simulink model "HT07PowertrainThermalModel3"  (R2022b)
(part 2 of 2)

  PS Gain : fl_lib/Physical Signals/Functions/PS Gain  gain=1
  PS Gain1 : fl_lib/Physical Signals/Functions/PS Gain  gain=2
  PS Gain2 : fl_lib/Physical Signals/Functions/PS Gain  gain=1
  PS Lookup Table (1D) : fl_lib/Physical Signals/Lookup Tables/PS Lookup Table (1D)  x=time  f=motorRearHeatGen J/s  interp_method=simscape.enum.interpolation.linear  extrap_method=simscape.enum.extrapolation.nearest
  PS Lookup Table (1D)1 : fl_lib/Physical Signals/Lookup Tables/PS Lookup Table (1D)  x=time  f=mcuHeatGen J/s  interp_method=simscape.enum.interpolation.linear  extrap_method=simscape.enum.extrapolation.nearest
  PS Lookup Table (1D)2 : fl_lib/Physical Signals/Lookup Tables/PS Lookup Table (1D)  x=time  f=velocity m/s  interp_method=simscape.enum.interpolation.linear  extrap_method=simscape.enum.extrapolation.nearest
  PS Lookup Table (1D)3 : fl_lib/Physical Signals/Lookup Tables/PS Lookup Table (1D)  Commented=on  x=time  f=velocity m/s  interp_method=simscape.enum.interpolation.linear  extrap_method=simscape.enum.extrapolation.nearest
  PS Lookup Table (1D)6 : fl_lib/Physical Signals/Lookup Tables/PS Lookup Table (1D)  Commented=on  x=time  f=velocity m/s  interp_method=simscape.enum.interpolation.linear  extrap_method=simscape.enum.extrapolation.nearest
  PS Lookup Table (1D)7 : fl_lib/Physical Signals/Lookup Tables/PS Lookup Table (1D)  x=time  f=motorFrontHeatGen J/s  interp_method=simscape.enum.interpolation.linear  extrap_method=simscape.enum.extrapolation.nearest
  PS Product : fl_lib/Physical Signals/Functions/PS Product
  PS Product1 : fl_lib/Physical Signals/Functions/PS Product  Commented=on
  PS Product2 : fl_lib/Physical Signals/Functions/PS Product  Commented=on
  PS Ramp{,1..2,5} (4 alike) : fl_lib/Physical Signals/Sources/PS Ramp  slope=1 1/s  start_time=0 s  initial_output=0
  PS Ramp3 : fl_lib/Physical Signals/Sources/PS Ramp  Commented=on  slope=1 1/s  start_time=0 s  initial_output=0
  PS Ramp4 : fl_lib/Physical Signals/Sources/PS Ramp  Commented=on  slope=1 1/s  start_time=0 s  initial_output=0
  PS-Simulink Converter{,5..8,11,31} (7 alike) : nesl_utility/PS-Simulink Converter  PhysicalDomain=network_engine_domain  SubClassName=ps_output  LeftPortType=input  RightPortType=output  PseudoPeriodic=off  Frequencies=[]  VectorFormat=inherit  Unit=inherit  AffineConversion=off
  PS-Simulink Converter1 : nesl_utility/PS-Simulink Converter  PhysicalDomain=network_engine_domain  SubClassName=ps_output  LeftPortType=input  RightPortType=output  PseudoPeriodic=off  Frequencies=[]  VectorFormat=1-D array  Unit=inherit  AffineConversion=off
  PS-Simulink Converter{3,9..10,13..18,20..30} (20 alike) : nesl_utility/PS-Simulink Converter  Commented=on  PhysicalDomain=network_engine_domain  SubClassName=ps_output  LeftPortType=input  RightPortType=output  PseudoPeriodic=off  Frequencies=[]  VectorFormat=inherit  Unit=inherit  AffineConversion=off
  PS-Simulink Converter12 : nesl_utility/PS-Simulink Converter  Commented=on  PhysicalDomain=network_engine_domain  SubClassName=ps_output  LeftPortType=input  RightPortType=output  PseudoPeriodic=off  Frequencies=[]  VectorFormat=1-D array  Unit=inherit  AffineConversion=off
  PS-Simulink Converter19 : nesl_utility/PS-Simulink Converter  Commented=on  PhysicalDomain=network_engine_domain  SubClassName=ps_output  LeftPortType=input  RightPortType=output  PseudoPeriodic=off  Frequencies=[]  VectorFormat=1-D array  Unit=inherit  AffineConversion=off
  PS-Simulink Converter2 : nesl_utility/PS-Simulink Converter  PhysicalDomain=network_engine_domain  SubClassName=ps_output  LeftPortType=input  RightPortType=output  PseudoPeriodic=off  Frequencies=[]  VectorFormat=1-D array  Unit=inherit  AffineConversion=off
  PS-Simulink Converter4 : nesl_utility/PS-Simulink Converter  PhysicalDomain=network_engine_domain  SubClassName=ps_output  LeftPortType=input  RightPortType=output  PseudoPeriodic=off  Frequencies=[]  VectorFormat=1-D array  Unit=inherit  AffineConversion=off
  PUMP TO MCU : fl_lib/Thermal Liquid/Elements/Pipe (TL)  Commented=on  length=tubeLengthPumpToMCU m  area=A m^2  Dh=d m  length_add=leqMCUToMotor m  roughness=tubeRoughness m  Re_lam=2000  Re_tur=4000  shape_factor=64  Nu_lam=3.66  dynamic_compressibility=simscape.enum.onoff.off  inertia=simscape.enum.onoff.off  p0=0.101325 MPa  T0=Tambient degC  mdot0=0 kg/s
  Perfect Insulator{,1..2,5} (4 alike) : fl_lib/Thermal/Thermal Elements/Perfect Insulator  T_specify=off  T_priority=None  T=0 K  T_nominal_specify=off  T_nominal_unit=K  T_nominal_value=1
  Perfect Insulator10 : fl_lib/Thermal/Thermal Elements/Perfect Insulator  Commented=on  T_specify=on  T_priority=High  T=Tambient degC  T_nominal_specify=off  T_nominal_unit=degC  T_nominal_value=Tambient
  Perfect Insulator12 : fl_lib/Thermal/Thermal Elements/Perfect Insulator  Commented=on  T_specify=off  T_priority=None  T=293.15 K  T_nominal_specify=off  T_nominal_unit=K  T_nominal_value=1
  Perfect Insulator13 : fl_lib/Thermal/Thermal Elements/Perfect Insulator  Commented=on  T_specify=off  T_priority=None  T=293.15 K  T_nominal_specify=off  T_nominal_unit=K  T_nominal_value=1
  Perfect Insulator14 : fl_lib/Thermal/Thermal Elements/Perfect Insulator  Commented=on  T_specify=off  T_priority=None  T=293.15 K  T_nominal_specify=off  T_nominal_unit=K  T_nominal_value=1
  Perfect Insulator{3,6,8..9} (4 alike) : fl_lib/Thermal/Thermal Elements/Perfect Insulator  Commented=on  T_specify=off  T_priority=None  T=0 K  T_nominal_specify=off  T_nominal_unit=K  T_nominal_value=1
  Perfect Insulator7 : fl_lib/Thermal/Thermal Elements/Perfect Insulator  Commented=on  T_specify=on  T_priority=High  T=Tambient degC  T_nominal_specify=off  T_nominal_unit=degC  T_nominal_value=Tambient
  Pipe (TL)1 : fl_lib/Thermal Liquid/Elements/Pipe (TL)  length=tubeLengthRadiatorToPump m  area=A m^2  Dh=d m  length_add=0 m  roughness=tubeRoughness m  Re_lam=2000  Re_tur=4000  shape_factor=64  Nu_lam=3.66  dynamic_compressibility=simscape.enum.onoff.off  inertia=simscape.enum.onoff.off  p0=0.101325 MPa  T0=Tamb degC  mdot0=0 kg/s
  Pipe (TL)2 : fl_lib/Thermal Liquid/Elements/Pipe (TL)  Commented=on  length=350 mm  area=A m^2  Dh=d m  length_add=0 m  roughness=tubeRoughness m  Re_lam=2000  Re_tur=4000  shape_factor=64  Nu_lam=3.66  dynamic_compressibility=simscape.enum.onoff.off  inertia=simscape.enum.onoff.off  p0=0.101325 MPa  T0=Tambient degC  mdot0=0 kg/s
  Pipe (TL)3 : fl_lib/Thermal Liquid/Elements/Pipe (TL)  length=tubeLengthMCUToMotor m  area=A m^2  Dh=d m  length_add=leqMCUToMotor m  roughness=tubeRoughness m  Re_lam=2000  Re_tur=4000  shape_factor=64  Nu_lam=3.66  dynamic_compressibility=simscape.enum.onoff.off  inertia=simscape.enum.onoff.off  p0=0.101325 MPa  T0=Tamb degC  mdot0=0 kg/s
  Pipe (TL)4 : fl_lib/Thermal Liquid/Elements/Pipe (TL)  length=tubeLengthMotorToRadiator m  area=A m^2  Dh=d m  length_add=leqMotorToRadiator m  roughness=tubeRoughness m  Re_lam=2000  Re_tur=4000  shape_factor=64  Nu_lam=3.66  dynamic_compressibility=simscape.enum.onoff.off  inertia=simscape.enum.onoff.off  p0=0.101325 MPa  T0=Tamb degC  mdot0=0 kg/s
  Pipe (TL)5 : fl_lib/Thermal Liquid/Elements/Pipe (TL)  length=tubeLengthPumpToMCU m  area=A m^2  Dh=d m  length_add=leqMCUToMotor m  roughness=tubeRoughness m  Re_lam=2000  Re_tur=4000  shape_factor=64  Nu_lam=3.66  dynamic_compressibility=simscape.enum.onoff.off  inertia=simscape.enum.onoff.off  p0=0.101325 MPa  T0=Tamb degC  mdot0=0 kg/s
  Pipe (TL)6 : fl_lib/Thermal Liquid/Elements/Pipe (TL)  Commented=on  length=210 mm  area=pi*((3/4)^2)/4 in^2  Dh=3/4 in  length_add=0 m  roughness=tubeRoughness m  Re_lam=2000  Re_tur=4000  shape_factor=64  Nu_lam=3.66  dynamic_compressibility=simscape.enum.onoff.off  inertia=simscape.enum.onoff.off  p0=0.101325 MPa  T0=Tambient degC  mdot0=0 kg/s
  Pipe (TL)7 : fl_lib/Thermal Liquid/Elements/Pipe (TL)  Commented=on  length=115 mm  area=pi*(0.5^2)/4 m^2  Dh=0.5 in  length_add=0 m  roughness=tubeRoughness m  Re_lam=2000  Re_tur=4000  shape_factor=64  Nu_lam=3.66  dynamic_compressibility=simscape.enum.onoff.off  inertia=simscape.enum.onoff.off  p0=0.101325 MPa  T0=Tambient degC  mdot0=0 kg/s
  Pressure & Temperature Sensor (TL){1..2,4..6,20} (6 alike) : fl_lib/Thermal Liquid/Sensors/Pressure & Temperature Sensor (TL)
      settings: InternalSimscapePortConfiguration="{\"Bottom\":[],\"Left\":[{\"id\":\"A\",\"label\":\"A\",\"type\":\"foundation.thermal_liquid.thermal_liquid\"}],\"Right\":[{\"id\":\"B\",\"label\":\"B\",\"type\":\"foundation.thermal_liquid.thermal_liquid\"},{\"id\":\"P\",\"label\":\"P\",\"type\":\"output\"},{\"id\":\"T\",\"label\":\"T\",\"type\":\"output\"}],\"Top\":[]}"
  Pressure & Temperature Sensor (TL){3,7..19} (14 alike) : fl_lib/Thermal Liquid/Sensors/Pressure & Temperature Sensor (TL)  Commented=on
      settings: InternalSimscapePortConfiguration="{\"Bottom\":[],\"Left\":[{\"id\":\"A\",\"label\":\"A\",\"type\":\"foundation.thermal_liquid.thermal_liquid\"}],\"Right\":[{\"id\":\"B\",\"label\":\"B\",\"type\":\"foundation.thermal_liquid.thermal_liquid\"},{\"id\":\"P\",\"label\":\"P\",\"type\":\"output\"},{\"id\":\"T\",\"label\":\"T\",\"type\":\"output\"}],\"Top\":[]}"
  Pressure Drop Across Pump : nesl_utility/PS-Simulink Converter  PhysicalDomain=network_engine_domain  SubClassName=ps_output  LeftPortType=input  RightPortType=output  PseudoPeriodic=off  Frequencies=[]  VectorFormat=1-D array  Unit=inherit  AffineConversion=off
  Pressures : Scope
  Product : Product
  Product1 : Product  Commented=on
  Product3 : Product  Commented=on
  RADIATOR TO SENSOR + SENSOR TO PUMP : fl_lib/Thermal Liquid/Elements/Pipe (TL)  Commented=on  length=47 in  area=0.0127^2/4*pi m^2  Dh=0.0127 m  length_add=0 m  roughness=tubeRoughness m  Re_lam=2000  Re_tur=4000  shape_factor=64  Nu_lam=3.66  dynamic_compressibility=simscape.enum.onoff.off  inertia=simscape.enum.onoff.off  p0=0.101325 MPa  T0=Tambient degC  mdot0=0 kg/s
  Radiator area [m^2]1 : Constant  Commented=on  Value=radiatorShroudArea
  Radiator area [m^2]2 : Constant  Commented=on  Value=radiatorShroudArea
  Radiator shroud area [m^2] : Constant  Value=radiator.ShroudArea
  Reservoir (G) : fl_lib/Gas/Elements/Reservoir (G)  pressure_spec=foundation.enum.pressure_spec.atmospheric  reservoir_pressure=0.101325 MPa  reservoir_temperature=Tamb degC  area_A=radiator.ShroudArea m^2
  Reservoir (G)1 : fl_lib/Gas/Elements/Reservoir (G)  pressure_spec=foundation.enum.pressure_spec.atmospheric  reservoir_pressure=0.101325 MPa  reservoir_temperature=Tamb degC  area_A=radiator.CoreArea m^2
  Reservoir (G)2 : fl_lib/Gas/Elements/Reservoir (G)  Commented=on  pressure_spec=foundation.enum.pressure_spec.atmospheric  reservoir_pressure=0.101325 MPa  reservoir_temperature=Tambient degC  area_A=radiatorShroudArea m^2
  Reservoir (G)3 : fl_lib/Gas/Elements/Reservoir (G)  Commented=on  pressure_spec=foundation.enum.pressure_spec.atmospheric  reservoir_pressure=0.101325 MPa  reservoir_temperature=Tambient degC  area_A=radiatorCoreArea m^2
  Reservoir (G)4 : fl_lib/Gas/Elements/Reservoir (G)  Commented=on  pressure_spec=foundation.enum.pressure_spec.atmospheric  reservoir_pressure=0.101325 MPa  reservoir_temperature=Tambient degC  area_A=radiatorShroudArea m^2
  Reservoir (G)5 : fl_lib/Gas/Elements/Reservoir (G)  Commented=on  pressure_spec=foundation.enum.pressure_spec.atmospheric  reservoir_pressure=0.101325 MPa  reservoir_temperature=Tambient degC  area_A=radiatorCoreArea m^2
  Scope{,2,5..8} (6 alike) : Scope  Commented=on
  Scope1 : Scope
  Scope3 : Scope  Commented=on  NumInputPorts=3
  Scope4 : Scope  Commented=on  NumInputPorts=3
  Sim Coolant Temp After MCU : Bias  Bias=-273  SaturateOnIntegerOverflow=off
  Sim Coolant Temp After Motor : Bias  Bias=-273  SaturateOnIntegerOverflow=off
  Sim Coolant Temp After Motor Front : Bias  Bias=-273  SaturateOnIntegerOverflow=off
  Sim Coolant Temp After Pump : Bias  Bias=-273  SaturateOnIntegerOverflow=off
  Sim Coolant Temp After Radiator : Bias  Bias=-273  SaturateOnIntegerOverflow=off
  Sim MCU Component Temp : nesl_utility/PS-Simulink Converter  PhysicalDomain=network_engine_domain  SubClassName=ps_output  LeftPortType=input  RightPortType=output  PseudoPeriodic=off  Frequencies=[]  VectorFormat=inherit  Unit=inherit  AffineConversion=off
  Sim Motor Front Temp : nesl_utility/PS-Simulink Converter  PhysicalDomain=network_engine_domain  SubClassName=ps_output  LeftPortType=input  RightPortType=output  PseudoPeriodic=off  Frequencies=[]  VectorFormat=1-D array  Unit=inherit  AffineConversion=off
  Sim Motor Rear Temp : nesl_utility/PS-Simulink Converter  PhysicalDomain=network_engine_domain  SubClassName=ps_output  LeftPortType=input  RightPortType=output  PseudoPeriodic=off  Frequencies=[]  VectorFormat=1-D array  Unit=inherit  AffineConversion=off
  Simulink-PS Converter1 : nesl_utility/Simulink-PS Converter  PhysicalDomain=network_engine_domain  SubClassName=ps_input  LeftPortType=input  RightPortType=output  PseudoPeriodic=off  Frequencies=[]  NoiseDistribution=none  NoiseParameters=[]  Unit=kg/m  AffineConversion=off  FilteringAndDerivatives=filter  SimscapeFilterOrder=1  InputFilterTimeConstant=0.01  UdotUserProvided=0
  Simulink-PS Converter2 : nesl_utility/Simulink-PS Converter  Commented=on  PhysicalDomain=network_engine_domain  SubClassName=ps_input  LeftPortType=input  RightPortType=output  PseudoPeriodic=off  Frequencies=[]  NoiseDistribution=none  NoiseParameters=[]  Unit=kg/m  AffineConversion=off  FilteringAndDerivatives=filter  SimscapeFilterOrder=1  InputFilterTimeConstant=0.01  UdotUserProvided=0
  Simulink-PS Converter4 : nesl_utility/Simulink-PS Converter  Commented=on  PhysicalDomain=network_engine_domain  SubClassName=ps_input  LeftPortType=input  RightPortType=output  PseudoPeriodic=off  Frequencies=[]  NoiseDistribution=none  NoiseParameters=[]  Unit=kg/m  AffineConversion=off  FilteringAndDerivatives=filter  SimscapeFilterOrder=1  InputFilterTimeConstant=0.01  UdotUserProvided=0
  Solver Configuration2 : nesl_utility/Solver Configuration  Commented=on  PhysicalDomain=network_engine_domain  SubClassName=solver  LeftPortType=input  RightPortType=generic  Tones=[]  Harmonics=[]  SimulateNoise=off  Profile=off  UseLocalSampling=off  EnableSwitchedLinearOptims=on  FrequencyDomain=off  UseCCode=off  RelTol=0.001  AbsTol=1e-06  MinStep=1e-09  ToWorkspace=off  RevertToSquareIcSolve=off  NumHomotopyIterations=100  PhasorMode=off  PhasorModeNumHarmonics=1  ConsistencySolver=NEWTON_FTOL  IndexReductionMethod=DerivativeReplacement  DoDC=off  ResidualTolerance=1e-08  ConsistencyTolSource=GLOBAL  ConsistencyAbsTol=0.001  ConsistencyRelTol=0.001  ConsistencyTolFactor=0.001  UseLocalSolver=off  LocalSolverChoice=NE_BACKWARD_EULER_ADVANCER  ResolveIndetEquations=on  FunctionEvalNumThread=1  LocalSolverSampleTime=0.001  DoFixedCost=off  MaxNonlinIter=3  MaxModeIter=2  ComputeImpulses=off  ImpulseIterations=2  LinearAlgebra=auto  LinearAlgebraNumThread=0  EquationFormulation=NE_TIME_EF  DelaysMemoryBudget=1024  AutomaticFiltering=on  FilteringTimeConstant=0.001  PartitionStorageMethod=AS_NEEDED  PartitionMemoryBudget=1024  PartitionMethod=ROBUST
  Solver Configuration3 : nesl_utility/Solver Configuration  PhysicalDomain=network_engine_domain  SubClassName=solver  LeftPortType=input  RightPortType=generic  Tones=[]  Harmonics=[]  SimulateNoise=off  Profile=off  UseLocalSampling=off  EnableSwitchedLinearOptims=on  FrequencyDomain=off  UseCCode=off  RelTol=0.001  AbsTol=1e-06  MinStep=1e-09  ToWorkspace=off  RevertToSquareIcSolve=off  NumHomotopyIterations=100  PhasorMode=off  PhasorModeNumHarmonics=1  ConsistencySolver=NEWTON_FTOL  IndexReductionMethod=DerivativeReplacement  DoDC=on  ResidualTolerance=1e-08  ConsistencyTolSource=GLOBAL  ConsistencyAbsTol=0.001  ConsistencyRelTol=0.001  ConsistencyTolFactor=0.001  UseLocalSolver=off  LocalSolverChoice=NE_BACKWARD_EULER_ADVANCER  ResolveIndetEquations=on  FunctionEvalNumThread=1  LocalSolverSampleTime=0.001  DoFixedCost=off  MaxNonlinIter=3  MaxModeIter=2  ComputeImpulses=off  ImpulseIterations=2  LinearAlgebra=auto  LinearAlgebraNumThread=0  EquationFormulation=NE_TIME_EF  DelaysMemoryBudget=1024  AutomaticFiltering=on  FilteringTimeConstant=0.001  PartitionStorageMethod=AS_NEEDED  PartitionMemoryBudget=1024  PartitionMethod=ROBUST
  Solver Configuration5 : nesl_utility/Solver Configuration  Commented=on  PhysicalDomain=network_engine_domain  SubClassName=solver  LeftPortType=input  RightPortType=generic  Tones=[]  Harmonics=[]  SimulateNoise=off  Profile=off  UseLocalSampling=off  EnableSwitchedLinearOptims=on  FrequencyDomain=off  UseCCode=off  RelTol=0.001  AbsTol=1e-06  MinStep=1e-09  ToWorkspace=off  RevertToSquareIcSolve=off  NumHomotopyIterations=100  PhasorMode=off  PhasorModeNumHarmonics=1  ConsistencySolver=NEWTON_FTOL  IndexReductionMethod=DerivativeReplacement  DoDC=off  ResidualTolerance=1e-08  ConsistencyTolSource=GLOBAL  ConsistencyAbsTol=0.001  ConsistencyRelTol=0.001  ConsistencyTolFactor=0.001  UseLocalSolver=off  LocalSolverChoice=NE_BACKWARD_EULER_ADVANCER  ResolveIndetEquations=on  FunctionEvalNumThread=1  LocalSolverSampleTime=0.001  DoFixedCost=off  MaxNonlinIter=3  MaxModeIter=2  ComputeImpulses=off  ImpulseIterations=2  LinearAlgebra=auto  LinearAlgebraNumThread=0  EquationFormulation=NE_TIME_EF  DelaysMemoryBudget=1024  AutomaticFiltering=on  FilteringTimeConstant=0.001  PartitionStorageMethod=AS_NEEDED  PartitionMemoryBudget=1024  PartitionMethod=ROBUST
  Tank (TL)1 : SimscapeFluids_lib/Thermal Liquid/Tanks & Accumulators/Tank (TL)  Commented=on  num_inlet=fluids.thermal_liquid.tanks_accumulators.enum.NumInlet.Two  pressure_spec=foundation.enum.pressure_spec.atmospheric  tank_pressure=0.101325 MPa  volume_spec=fluids.thermal_liquid.tanks_accumulators.enum.TankVolumeSpec.Constant  tank_area=0.005 m^2  level_TLU=[0, 3, 5] m  volume_TLU=[0, 4, 6] m^3  inlet_height_A=0.1 m  inlet_area_A=0.01 m^2  inlet_heights_AB=[0, 0] m  inlet_areas_AB=[.01, .01] m^2  inlet_heights_ABC=[.1, .1, .1] m  inlet_areas_ABC=[.01, .01, .01] m^2  inlet_heights_ABCD=0.1 * ones(1, 4) m  inlet_areas_ABCD=0.01 * ones(1, 4) m^2  inlet_heights_ABCDE=0.1 * ones(1, 5) m  inlet_areas_ABCDE=0.01 * ones(1, 5) m^2  inlet_heights_ABCDEF=0.1 * ones(1, 6) m  inlet_areas_ABCDEF=0.01 * ones(1, 6) m^2  level_check=simscape.enum.assert.action.none  capacity_check=simscape.enum.assert.action.error  max_capacity=1 l  g=9.81 m/s^2  level_specify=on  level_priority=High  level=0.05 m  level_nominal_specify=off  level_nominal_unit=m  level_nominal_value=1  volume_specify=on  volume_priority=High  volume=0.5 l  volume_nominal_specify=off  volume_nominal_unit=m^3  volume_nominal_value=1  mass_specify=off  mass_priority=None  mass=5000 kg  mass_nominal_specify=off  mass_nominal_unit=kg  mass_nominal_value=1  T_I_specify=on  T_I_priority=High  T_I=Tamb degC  T_I_nominal_specify=off  T_I_nominal_unit=K  T_I_nominal_value=1
      settings: InternalSimscapePortConfiguration="{\"Bottom\":[{\"id\":\"H\",\"label\":\"H\",\"type\":\"foundation.thermal.thermal\"},{\"id\":\"T_out\",\"label\":\"T\",\"type\":\"output\"}],\"Left\":[{\"id\":\"A\",\"label\":\"A\",\"type\":\"foundation.thermal_liquid.thermal_liquid\"},{\"id\":\"B\",\"label\":\"B\",\"type\":\"foundation.thermal_liquid.thermal_liquid\"}],\"Right\":[],\"Top\":[{\"id\":\"V_out\",\"label\":\"V\",\"type\":\"output\"},{\"id\":\"L_out\",\"label\":\"L\",\"type\":\"output\"}]}"
  Tank (TL)2 : SimscapeFluids_lib/Thermal Liquid/Tanks & Accumulators/Tank (TL)  Commented=on  num_inlet=fluids.thermal_liquid.tanks_accumulators.enum.NumInlet.Two  pressure_spec=foundation.enum.pressure_spec.atmospheric  tank_pressure=0.101325 MPa  volume_spec=fluids.thermal_liquid.tanks_accumulators.enum.TankVolumeSpec.Constant  tank_area=0.005 m^2  level_TLU=[0, 3, 5] m  volume_TLU=[0, 4, 6] m^3  inlet_height_A=0.1 m  inlet_area_A=0.01 m^2  inlet_heights_AB=[0, 0] m  inlet_areas_AB=[.01, .01] m^2  inlet_heights_ABC=[.1, .1, .1] m  inlet_areas_ABC=[.01, .01, .01] m^2  inlet_heights_ABCD=0.1 * ones(1, 4) m  inlet_areas_ABCD=0.01 * ones(1, 4) m^2  inlet_heights_ABCDE=0.1 * ones(1, 5) m  inlet_areas_ABCDE=0.01 * ones(1, 5) m^2  inlet_heights_ABCDEF=0.1 * ones(1, 6) m  inlet_areas_ABCDEF=0.01 * ones(1, 6) m^2  level_check=simscape.enum.assert.action.none  capacity_check=simscape.enum.assert.action.error  max_capacity=1 l  g=9.81 m/s^2  level_specify=on  level_priority=High  level=0.05 m  level_nominal_specify=off  level_nominal_unit=m  level_nominal_value=1  volume_specify=on  volume_priority=High  volume=0.5 l  volume_nominal_specify=off  volume_nominal_unit=m^3  volume_nominal_value=1  mass_specify=off  mass_priority=None  mass=5000 kg  mass_nominal_specify=off  mass_nominal_unit=kg  mass_nominal_value=1  T_I_specify=on  T_I_priority=High  T_I=Tamb degC  T_I_nominal_specify=off  T_I_nominal_unit=K  T_I_nominal_value=1
      settings: InternalSimscapePortConfiguration="{\"Bottom\":[{\"id\":\"H\",\"label\":\"H\",\"type\":\"foundation.thermal.thermal\"},{\"id\":\"T_out\",\"label\":\"T\",\"type\":\"output\"}],\"Left\":[{\"id\":\"A\",\"label\":\"A\",\"type\":\"foundation.thermal_liquid.thermal_liquid\"},{\"id\":\"B\",\"label\":\"B\",\"type\":\"foundation.thermal_liquid.thermal_liquid\"}],\"Right\":[],\"Top\":[{\"id\":\"V_out\",\"label\":\"V\",\"type\":\"output\"},{\"id\":\"L_out\",\"label\":\"L\",\"type\":\"output\"}]}"
  Tank (TL)3 : SimscapeFluids_lib/Thermal Liquid/Tanks & Accumulators/Tank (TL)  num_inlet=fluids.thermal_liquid.tanks_accumulators.enum.NumInlet.Two  pressure_spec=foundation.enum.pressure_spec.atmospheric  tank_pressure=0.101325 MPa  volume_spec=fluids.thermal_liquid.tanks_accumulators.enum.TankVolumeSpec.Constant  tank_area=radiator.effectiveCrossSection m^2  level_TLU=[0, 3, 5] m  volume_TLU=[0, 4, 6] m^3  inlet_height_A=0.1 m  inlet_area_A=0.01 m^2  inlet_heights_AB=[0, 0] m  inlet_areas_AB=[.01, .01] m^2  inlet_heights_ABC=[.1, .1, .1] m  inlet_areas_ABC=[.01, .01, .01] m^2  inlet_heights_ABCD=0.1 * ones(1, 4) m  inlet_areas_ABCD=0.01 * ones(1, 4) m^2  inlet_heights_ABCDE=0.1 * ones(1, 5) m  inlet_areas_ABCDE=0.01 * ones(1, 5) m^2  inlet_heights_ABCDEF=0.1 * ones(1, 6) m  inlet_areas_ABCDEF=0.01 * ones(1, 6) m^2  level_check=simscape.enum.assert.action.none  capacity_check=simscape.enum.assert.action.error  max_capacity=2*radiator.waterVolumeL l  g=9.81 m/s^2  level_specify=on  level_priority=High  level=radiator.CoreHeight m  level_nominal_specify=off  level_nominal_unit=m  level_nominal_value=1  volume_specify=on  volume_priority=High  volume=radiator.waterVolumeL l  volume_nominal_specify=off  volume_nominal_unit=m^3  volume_nominal_value=1  mass_specify=off  mass_priority=None  mass=5000 kg  mass_nominal_specify=off  mass_nominal_unit=kg  mass_nominal_value=1  T_I_specify=on  T_I_priority=High  T_I=Tamb degC  T_I_nominal_specify=off  T_I_nominal_unit=K  T_I_nominal_value=1
      settings: InternalSimscapePortConfiguration="{\"Bottom\":[{\"id\":\"H\",\"label\":\"H\",\"type\":\"foundation.thermal.thermal\"},{\"id\":\"T_out\",\"label\":\"T\",\"type\":\"output\"}],\"Left\":[{\"id\":\"A\",\"label\":\"A\",\"type\":\"foundation.thermal_liquid.thermal_liquid\"},{\"id\":\"B\",\"label\":\"B\",\"type\":\"foundation.thermal_liquid.thermal_liquid\"}],\"Right\":[],\"Top\":[{\"id\":\"V_out\",\"label\":\"V\",\"type\":\"output\"},{\"id\":\"L_out\",\"label\":\"L\",\"type\":\"output\"}]}"
  Temperature Sensor : fl_lib/Thermal/Thermal Sensors/Temperature Sensor
  Temperature Source : fl_lib/Thermal/Thermal Sources/Temperature Source  temperature=0 degC
  Temperature Source1 : fl_lib/Thermal/Thermal Sources/Temperature Source  temperature=0 degC
  Temperature Source3 : fl_lib/Thermal/Thermal Sources/Temperature Source  temperature=0 degC
  Temperatures : Scope  NumInputPorts=5
  Thermal Liquid Properties (TL)1 : SimscapeFluids_lib/Thermal Liquid/Utilities/Thermal Liquid Properties (TL)  fluid_list=fluids.thermal_liquid.utilities.enum.thermal_liquid_fluid_list.water  concentration_param_EG=fluids.thermal_liquid.utilities.enum.thermal_liquid_concentration.volume_fraction  concentration_param_PG=fluids.thermal_liquid.utilities.enum.thermal_liquid_concentration.volume_fraction  c_mass_SW=3.5e-3  c_mass_EG=0.1  c_mass_PG=0.1  c_mass_GL=0.1  c_vol_EG=0.1  c_vol_PG=0.1  beta_const_EG=2.1791 GPa  beta_const_PG=2.1791 GPa  beta_const_GL=2.1791 GPa  p_min_EG=0.01 MPa  p_min_PG=0.01 MPa  p_min_GL=0.01 MPa  p_max_EG=50 MPa  p_max_PG=50 MPa  p_max_GL=50 MPa  p_atm=0.101325 MPa
  Thermal Liquid Properties (TL)2 : SimscapeFluids_lib/Thermal Liquid/Utilities/Thermal Liquid Properties (TL)  Commented=on  fluid_list=fluids.thermal_liquid.utilities.enum.thermal_liquid_fluid_list.water  concentration_param_EG=fluids.thermal_liquid.utilities.enum.thermal_liquid_concentration.volume_fraction  concentration_param_PG=fluids.thermal_liquid.utilities.enum.thermal_liquid_concentration.volume_fraction  c_mass_SW=3.5e-3  c_mass_EG=0.1  c_mass_PG=0.1  c_mass_GL=0.1  c_vol_EG=0.1  c_vol_PG=0.1  beta_const_EG=2.1791 GPa  beta_const_PG=2.1791 GPa  beta_const_GL=2.1791 GPa  p_min_EG=0.01 MPa  p_min_PG=0.01 MPa  p_min_GL=0.01 MPa  p_max_EG=50 MPa  p_max_PG=50 MPa  p_max_GL=50 MPa  p_atm=0.101325 MPa
  Thermal Liquid Properties (TL)3 : SimscapeFluids_lib/Thermal Liquid/Utilities/Thermal Liquid Properties (TL)  Commented=on  fluid_list=fluids.thermal_liquid.utilities.enum.thermal_liquid_fluid_list.water  concentration_param_EG=fluids.thermal_liquid.utilities.enum.thermal_liquid_concentration.volume_fraction  concentration_param_PG=fluids.thermal_liquid.utilities.enum.thermal_liquid_concentration.volume_fraction  c_mass_SW=3.5e-3  c_mass_EG=0.1  c_mass_PG=0.1  c_mass_GL=0.1  c_vol_EG=0.1  c_vol_PG=0.1  beta_const_EG=2.1791 GPa  beta_const_PG=2.1791 GPa  beta_const_GL=2.1791 GPa  p_min_EG=0.01 MPa  p_min_PG=0.01 MPa  p_min_GL=0.01 MPa  p_max_EG=50 MPa  p_max_PG=50 MPa  p_max_GL=50 MPa  p_atm=0.101325 MPa
  Thermal Mass : fl_lib/Thermal/Thermal Elements/Thermal Mass  mass=coldPlateMassMCU kg  sp_heat=cAl J/(K*kg)  num_ports=foundation.enum.numPorts2.one  T_specify=on  T_priority=High  T=Tamb degC  T_nominal_specify=off  T_nominal_unit=K  T_nominal_value=1  Q_specify=off  Q_priority=None  Q=0 W  Q_nominal_specify=off  Q_nominal_unit=W  Q_nominal_value=1
  Thermal Mass1 : fl_lib/Thermal/Thermal Elements/Thermal Mass  Commented=on  mass=radiator.Mass kg  sp_heat=cAl J/(K*kg)  num_ports=foundation.enum.numPorts2.one  T_specify=on  T_priority=High  T=Tamb degC  T_nominal_specify=off  T_nominal_unit=K  T_nominal_value=Tamb + 273.15  Q_specify=off  Q_priority=None  Q=0 W  Q_nominal_specify=off  Q_nominal_unit=W  Q_nominal_value=1
  Thermal Reference : fl_lib/Thermal/Thermal Elements/Thermal Reference
  Thermal Reference1 : fl_lib/Thermal/Thermal Elements/Thermal Reference
  Thermal Reference2 : fl_lib/Thermal/Thermal Elements/Thermal Reference
  head : Scope  Commented=on  NumInputPorts=3
  head1 : Scope  Commented=on  NumInputPorts=3
  pump : Gain  Commented=on  Gain=0.000102
  pump1 : Gain  Commented=on  Gain=0.000102
  radiator : Gain  Commented=on  Gain=0.000102
  radiator1 : Gain  Commented=on  Gain=0.000102
  reservoir : Gain  Commented=on  Gain=0.000102
  reservoir1 : Gain  Commented=on  Gain=0.000102
  wires:
  Radiator shroud area [m^2]/1 -> Product/2
  Product/1 -> Simulink-PS Converter1/1
  Air density [kg/m^3]/1 -> Product/1
  Pressure Drop Across Pump/1 -> Pressures/1
  Sim MCU Component Temp/1 -> Temperatures/1
  Integrator1/1 -> MCU Heat Gen Scope/1
  PS-Simulink Converter7/1 -> Integrator1/1
  PS-Simulink Converter6/1 -> Sim Coolant Temp After Radiator/1
  PS-Simulink Converter11/1 -> Scope1/1
  Gain/1 -> Mass Flow Rate/1
  PS-Simulink Converter2/1 -> Gain/1
  Radiator area [m^2]1/1 -> Product1/2
  Product1/1 -> Simulink-PS Converter2/1
  Air density [kg/m^3]1/1 -> Product1/1
  PS-Simulink Converter12/1 -> Gain1/1
  Gain1/1 -> Mass Flow Rate1/1
  Sim Coolant Temp After Radiator/1 -> Coolant Water Temperatures/5, Temperatures/2
  PS-Simulink Converter/1 -> Sim Coolant Temp After Pump/1
  PS-Simulink Converter5/1 -> Sim Coolant Temp After MCU/1
  PS-Simulink Converter8/1 -> Sim Coolant Temp After Motor/1
  Sim Coolant Temp After Pump/1 -> Coolant Water Temperatures/4
  Sim Coolant Temp After MCU/1 -> Coolant Water Temperatures/3
  Sim Coolant Temp After Motor/1 -> Coolant Water Temperatures/1
  pump/1 -> head/1
  PS-Simulink Converter3/1 -> radiator/1
  PS-Simulink Converter10/1 -> pump/1
  radiator/1 -> head/2
  PS-Simulink Converter9/1 -> reservoir/1
  reservoir/1 -> head/3
  PS-Simulink Converter15/1 -> Add Constant/1
  Add Constant/1 -> Scope3/1
  PS-Simulink Converter16/1 -> Add Constant1/1
  Add Constant1/1 -> Scope3/3
  PS-Simulink Converter17/1 -> Absolute Pressure/1
  PS-Simulink Converter18/1 -> Add Constant2/1
  Add Constant2/1 -> Scope3/2
  PS-Simulink Converter25/1 -> Scope8/1
  PS-Simulink Converter24/1 -> Scope7/1
  PS-Simulink Converter13/1 -> Scope/1
  PS-Simulink Converter29/1 -> radiator1/1
  PS-Simulink Converter22/1 -> Add Constant4/1
  PS-Simulink Converter21/1 -> Add Constant3/1
  Add Constant4/1 -> Scope4/3
  PS-Simulink Converter27/1 -> Scope5/1
  PS-Simulink Converter28/1 -> Scope6/1
  pump1/1 -> head1/1
  PS-Simulink Converter30/1 -> reservoir1/1
  Air density [kg/m^3]2/1 -> Product3/1
  Product3/1 -> Simulink-PS Converter4/1
  Add Constant3/1 -> Scope4/1
  PS-Simulink Converter26/1 -> Add Constant5/1
  Radiator area [m^2]2/1 -> Product3/2
  PS-Simulink Converter23/1 -> Absolute Pressure1/1
  reservoir1/1 -> head1/3
  Add Constant5/1 -> Scope4/2
  PS-Simulink Converter20/1 -> Scope2/1
  PS-Simulink Converter14/1 -> pump1/1
  radiator1/1 -> head1/2
  PS-Simulink Converter19/1 -> Gain2/1
  Gain2/1 -> Mass Flow Rate2/1
  MOTOR PRESSURE DROP/1 -> MOTOR AND MCU PRESSURE DROP/1
  MCU PRESSURE DROP/1 -> MOTOR AND MCU PRESSURE DROP/2
  PS-Simulink Converter1/1 -> Integrator/1
  Integrator/1 -> MotorRear Gen Scope/1
  Integrator2/1 -> MotorFront Heat Gen/1
  PS-Simulink Converter4/1 -> Integrator2/1
  Sim Motor Front Temp/1 -> Temperatures/4
  Sim Motor Rear Temp/1 -> Temperatures/5
  PS-Simulink Converter31/1 -> Sim Coolant Temp After Motor Front/1
  Sim Coolant Temp After Motor Front/1 -> Coolant Water Temperatures/2
  connections:
  Thermal Reference1/LConn1 -- Controlled Heat Flow Rate Source1/RConn2
  PS Lookup Table (1D)1/RConn1 -- PS Gain1/LConn1
  PS Ramp2/RConn1 -- PS Lookup Table (1D)1/LConn1
  Gas Properties (G)/RConn1 -- Heat Exchanger (G-TL)3/LConn2 -- Controlled Mass Flow Rate Source (G)/RConn1
  MCU COOLER HT06/LConn2 -- Temperature Sensor/LConn1 -- Thermal Mass/LConn1 -- Heat Flow Rate Sensor1/RConn2
  Heat Exchanger (G-TL)3/LConn1 -- Reservoir (G)1/LConn1
  Reservoir (G)/LConn1 -- Controlled Mass Flow Rate Source (G)/LConn1
  Ideal Angular Velocity Source/RConn2 -- Centrifugal Pump (TL)/RConn2 -- Mechanical Rotational Reference/LConn1
  PS Constant/RConn1 -- Ideal Angular Velocity Source/RConn1
  Perfect Insulator/LConn1 -- Pipe (TL)1/LConn2
  Pipe (TL)1/RConn1 -- Pressure & Temperature Sensor (TL)2/LConn1 -- Pressure & Temperature Sensor (TL)5/RConn1 -- Centrifugal Pump (TL)/LConn1
  Mass & Energy Flow Rate Sensor (TL)/LConn1 -- Pressure & Temperature Sensor (TL)5/LConn1 -- Centrifugal Pump (TL)/LConn2 -- Thermal Liquid Properties (TL)1/RConn1 -- Solver Configuration3/RConn1
  PS-Simulink Converter2/LConn1 -- Mass & Energy Flow Rate Sensor (TL)/RConn2
  Absolute Reference (TL)3/LConn1 -- Pressure & Temperature Sensor (TL)2/RConn1
  Pressure & Temperature Sensor (TL)2/RConn3 -- PS-Simulink Converter6/LConn1
  Controlled Heat Flow Rate Source1/LConn1 -- Heat Flow Rate Sensor1/LConn1
  Heat Flow Rate Sensor1/RConn1 -- PS-Simulink Converter7/LConn1
  Temperature Source/LConn1 -- Temperature Sensor/RConn1
  Perfect Insulator1/LConn1 -- Pipe (TL)3/LConn2
  Pipe (TL)4/LConn2 -- Perfect Insulator2/LConn1
  PS Ramp1/RConn1 -- PS Lookup Table (1D)2/LConn1
  PS Product/RConn1 -- Aerodynamic Adjuster/LConn1
  PS Product/LConn1 -- PS Lookup Table (1D)2/RConn1
  PS Product/LConn2 -- Simulink-PS Converter1/RConn1
  Perfect Insulator5/LConn1 -- Pipe (TL)5/LConn2
  Ideal Angular Velocity Source/LConn1 -- Centrifugal Pump (TL)/RConn1
  Mechanical Rotational Reference1/LConn1 -- Ideal Angular Velocity Source1/RConn2 -- Centrifugal Pump (TL)1/RConn2
  PS Constant1/RConn1 -- Ideal Angular Velocity Source1/RConn1
  Centrifugal Pump (TL)1/RConn1 -- Ideal Angular Velocity Source1/LConn1
  Controlled Mass Flow Rate Source (G)1/RConn1 -- Heat Exchanger (G-TL)1/LConn2 -- Gas Properties (G)1/RConn1
  PS Product1/RConn1 -- PS-Simulink Converter13/LConn1 -- Controlled Mass Flow Rate Source (G)1/LConn2
  Heat Exchanger (G-TL)1/LConn1 -- Reservoir (G)3/LConn1
  Reservoir (G)2/LConn1 -- Controlled Mass Flow Rate Source (G)1/LConn1
  PS Product1/LConn1 -- PS Lookup Table (1D)3/RConn1
  PS Product1/LConn2 -- Simulink-PS Converter2/RConn1
  PS Ramp3/RConn1 -- PS Lookup Table (1D)3/LConn1
  Thermal Liquid Properties (TL)2/RConn1 -- Pipe (TL)6/LConn1 -- Tank (TL)1/LConn2 -- Pressure & Temperature Sensor (TL)8/RConn1 -- Pressure & Temperature Sensor (TL)9/LConn1
  PS-Simulink Converter12/LConn1 -- Mass & Energy Flow Rate Sensor (TL)1/RConn2
  Mass & Energy Flow Rate Sensor (TL)1/LConn1 -- Centrifugal Pump (TL)1/LConn2
  Pressure & Temperature Sensor (TL)11/LConn1 -- Heat Exchanger (G-TL)1/RConn1 -- Pressure & Temperature Sensor (TL)3/RConn1 -- Tank (TL)1/LConn1 -- Pressure & Temperature Sensor (TL)8/LConn1
  Perfect Insulator9/LConn1 -- Pipe (TL)7/LConn2
  Heat Exchanger (G-TL)3/RConn2 -- Pipe (TL)4/RConn1
  Pipe (TL)1/LConn1 -- Tank (TL)3/LConn2
  Pipe (TL)5/LConn1 -- Mass & Energy Flow Rate Sensor (TL)/RConn1
  Pipe (TL)4/LConn1 -- MOTOR COOLER REAR/RConn1 -- Pressure & Temperature Sensor (TL)6/LConn1
  Pipe (TL)5/RConn1 -- Pressure & Temperature Sensor (TL)1/LConn1 -- MCU COOLER HT06/LConn1
  Pipe (TL)3/LConn1 -- MCU COOLER HT06/RConn1 -- Pressure & Temperature Sensor (TL)4/LConn1
  Pressure Drop Across Pump/LConn1 -- Pressure & Temperature Sensor (TL)5/RConn2
  Sim MCU Component Temp/LConn1 -- Temperature Sensor/RConn2
  Aerodynamic Adjuster/RConn1 -- PS-Simulink Converter11/LConn1 -- Controlled Mass Flow Rate Source (G)/LConn2
  Absolute Reference (TL)1/LConn1 -- Pressure & Temperature Sensor (TL)1/RConn1
  PS-Simulink Converter/LConn1 -- Pressure & Temperature Sensor (TL)1/RConn3
  Absolute Reference (TL)2/LConn1 -- Pressure & Temperature Sensor (TL)4/RConn1
  PS-Simulink Converter5/LConn1 -- Pressure & Temperature Sensor (TL)4/RConn3
  Absolute Reference (TL)4/LConn1 -- Pressure & Temperature Sensor (TL)6/RConn1
  PS-Simulink Converter8/LConn1 -- Pressure & Temperature Sensor (TL)6/RConn3
  Pressure & Temperature Sensor (TL)3/RConn2 -- PS-Simulink Converter3/LConn1
  Pressure & Temperature Sensor (TL)7/RConn2 -- PS-Simulink Converter10/LConn1
  Pressure & Temperature Sensor (TL)8/RConn2 -- PS-Simulink Converter9/LConn1
  Absolute Reference (TL)/LConn1 -- Pressure & Temperature Sensor (TL)9/RConn1
  Pressure & Temperature Sensor (TL)9/RConn3 -- PS-Simulink Converter15/LConn1
  Absolute Reference (TL)5/LConn1 -- Pressure & Temperature Sensor (TL)10/RConn1
  Pressure & Temperature Sensor (TL)10/RConn3 -- PS-Simulink Converter16/LConn1
  Pressure & Temperature Sensor (TL)9/RConn2 -- PS-Simulink Converter17/LConn1
  Pressure & Temperature Sensor (TL)11/RConn1 -- Absolute Reference (TL)6/LConn1
  Pressure & Temperature Sensor (TL)11/RConn3 -- PS-Simulink Converter18/LConn1
  PS-Simulink Converter24/LConn1 -- Tank (TL)1/RConn2
  Perfect Insulator10/LConn1 -- Tank (TL)1/RConn1
  PS-Simulink Converter25/LConn1 -- Tank (TL)1/LConn4
  Solver Configuration2/RConn1 -- Pipe (TL)7/RConn1 -- Pressure & Temperature Sensor (TL)7/RConn1 -- Mass & Energy Flow Rate Sensor (TL)1/RConn1
  Perfect Insulator6/LConn1 -- Pipe (TL)6/LConn2
  Centrifugal Pump (TL)1/LConn1 -- Pressure & Temperature Sensor (TL)7/LConn1 -- Pipe (TL)6/RConn1
  Pressure & Temperature Sensor (TL)16/LConn1 -- Tank (TL)2/LConn1 -- Heat Exchanger (G-TL)2/RConn1 -- Pressure & Temperature Sensor (TL)13/LConn1 -- Pressure & Temperature Sensor (TL)14/RConn1
  Pressure & Temperature Sensor (TL)14/LConn1 -- Heat Exchanger (G-TL)2/RConn2 -- Pressure & Temperature Sensor (TL)12/LConn1 -- MOTOR TO RADIATOR/RConn1
  Pressure & Temperature Sensor (TL)15/LConn1 -- Centrifugal Pump (TL)2/LConn1 -- RADIATOR TO SENSOR + SENSOR TO PUMP/RConn1
  Pressure & Temperature Sensor (TL)17/LConn1 -- Solver Configuration5/RConn1 -- Tank (TL)2/LConn2 -- Pressure & Temperature Sensor (TL)16/RConn1 -- Thermal Liquid Properties (TL)3/RConn1 -- RADIATOR TO SENSOR + SENSOR TO PUMP/LConn1
  Controlled Mass Flow Rate Source (G)2/LConn2 -- PS-Simulink Converter20/LConn1 -- PS Product2/RConn1
  Gas Properties (G)2/RConn1 -- Heat Exchanger (G-TL)2/LConn2 -- Controlled Mass Flow Rate Source (G)2/RConn1
  Mechanical Rotational Reference2/LConn1 -- Ideal Angular Velocity Source2/RConn2 -- Centrifugal Pump (TL)2/RConn2
  Pressure & Temperature Sensor (TL)12/RConn3 -- PS-Simulink Converter22/LConn1
  Heat Exchanger (G-TL)2/LConn1 -- Reservoir (G)5/LConn1
  PS Ramp4/RConn1 -- PS Lookup Table (1D)6/LConn1
  Pressure & Temperature Sensor (TL)17/RConn3 -- PS-Simulink Converter21/LConn1
  PS-Simulink Converter28/LConn1 -- Tank (TL)2/LConn4
  Pressure & Temperature Sensor (TL)15/RConn2 -- PS-Simulink Converter14/LConn1
  PS-Simulink Converter19/LConn1 -- Mass & Energy Flow Rate Sensor (TL)2/RConn2
  Mass & Energy Flow Rate Sensor (TL)2/LConn1 -- Pressure & Temperature Sensor (TL)15/RConn1 -- Centrifugal Pump (TL)2/LConn2
  Pressure & Temperature Sensor (TL)13/RConn1 -- Absolute Reference (TL)9/LConn1
  Pressure & Temperature Sensor (TL)14/RConn2 -- PS-Simulink Converter29/LConn1
  Perfect Insulator7/LConn1 -- Tank (TL)2/RConn1
  PS Product2/LConn1 -- PS Lookup Table (1D)6/RConn1
  PS-Simulink Converter27/LConn1 -- Tank (TL)2/RConn2
  Reservoir (G)4/LConn1 -- Controlled Mass Flow Rate Source (G)2/LConn1
  Pressure & Temperature Sensor (TL)13/RConn3 -- PS-Simulink Converter26/LConn1
  Pressure & Temperature Sensor (TL)17/RConn2 -- PS-Simulink Converter23/LConn1
  Absolute Reference (TL)7/LConn1 -- Pressure & Temperature Sensor (TL)17/RConn1
  PS Product2/LConn2 -- Simulink-PS Converter4/RConn1
  Absolute Reference (TL)8/LConn1 -- Pressure & Temperature Sensor (TL)12/RConn1
  Perfect Insulator8/LConn1 -- RADIATOR TO SENSOR + SENSOR TO PUMP/LConn2
  PS Constant2/RConn1 -- Ideal Angular Velocity Source2/RConn1
  Centrifugal Pump (TL)2/RConn1 -- Ideal Angular Velocity Source2/LConn1
  Pressure & Temperature Sensor (TL)16/RConn2 -- PS-Simulink Converter30/LConn1
  PUMP TO MCU/RConn1 -- Pressure & Temperature Sensor (TL)19/LConn1 -- MCU COOLER/LConn1
  MCU COOLER/RConn1 -- Pressure & Temperature Sensor (TL)19/RConn1 -- MCU TO MOTOR/LConn1
  MOTOR COOLER/LConn1 -- Pressure & Temperature Sensor (TL)18/LConn1 -- MCU TO MOTOR/RConn1
  MOTOR COOLER/RConn1 -- MOTOR TO RADIATOR/LConn1 -- Pressure & Temperature Sensor (TL)18/RConn1
  Motor Thermal Mass1/LConn1 -- MOTOR COOLER/LConn2
  Perfect Insulator13/LConn1 -- MCU COOLER/LConn2
  Perfect Insulator12/LConn1 -- MCU TO MOTOR/LConn2
  Perfect Insulator14/LConn1 -- MOTOR TO RADIATOR/LConn2
  PUMP TO MCU/LConn1 -- Mass & Energy Flow Rate Sensor (TL)2/RConn1
  Pressure & Temperature Sensor (TL)18/RConn2 -- MOTOR PRESSURE DROP/LConn1
  MCU PRESSURE DROP/LConn1 -- Pressure & Temperature Sensor (TL)19/RConn2
  Heat Exchanger (G-TL)3/RConn1 -- Tank (TL)3/LConn1
  Controlled Heat Flow Rate Source1/RConn1 -- PS Gain1/RConn1
  Pressure & Temperature Sensor (TL)3/LConn1 -- Heat Exchanger (G-TL)1/RConn2 -- Pipe (TL)2/LConn1
  Pipe (TL)7/LConn1 -- Pipe (TL)2/RConn1 -- Pressure & Temperature Sensor (TL)10/LConn1
  Perfect Insulator3/LConn1 -- Pipe (TL)2/LConn2
  MOTOR COOLER REAR/LConn2 -- MotorRear Temperature Sensor/LConn1 -- Heat Flow Rate Sensor/RConn2 -- MotorRear Thermal Mass/LConn1
  Heat Flow Rate Sensor2/RConn2 -- MOTOR COOLER FRONT/LConn2 -- MotorFront Temperature Sensor/LConn1 -- MotorFront Thermal Mass/LConn1
  PS Lookup Table (1D)/RConn1 -- PS Gain/LConn1
  Controlled Heat Flow Rate Source/LConn1 -- Heat Flow Rate Sensor/LConn1
  Thermal Reference/LConn1 -- Controlled Heat Flow Rate Source/RConn2
  Heat Flow Rate Sensor/RConn1 -- PS-Simulink Converter1/LConn1
  PS Ramp/RConn1 -- PS Lookup Table (1D)/LConn1
  PS Lookup Table (1D)7/RConn1 -- PS Gain2/LConn1
  Heat Flow Rate Sensor2/RConn1 -- PS-Simulink Converter4/LConn1
  Temperature Source3/LConn1 -- MotorFront Temperature Sensor/RConn1
  PS Gain2/RConn1 -- Controlled Heat Flow Rate Source2/RConn1
  PS Ramp5/RConn1 -- PS Lookup Table (1D)7/LConn1
  PS Gain/RConn1 -- Controlled Heat Flow Rate Source/RConn1
  Thermal Reference2/LConn1 -- Controlled Heat Flow Rate Source2/RConn2
  Controlled Heat Flow Rate Source2/LConn1 -- Heat Flow Rate Sensor2/LConn1
  Temperature Source1/LConn1 -- MotorRear Temperature Sensor/RConn1
  MotorRear Temperature Sensor/RConn2 -- Sim Motor Rear Temp/LConn1
  MotorFront Temperature Sensor/RConn2 -- Sim Motor Front Temp/LConn1
  Thermal Mass1/LConn1 -- Tank (TL)3/RConn1
  Pressure & Temperature Sensor (TL)20/LConn1 -- MOTOR COOLER FRONT/RConn1 -- MOTOR COOLER REAR/LConn1
  MOTOR COOLER FRONT/LConn1 -- Pipe (TL)3/RConn1
  PS-Simulink Converter31/LConn1 -- Pressure & Temperature Sensor (TL)20/RConn3
  Absolute Reference (TL)10/LConn1 -- Pressure & Temperature Sensor (TL)20/RConn1
